simulink model "Code_Gene_Electronic_Throttle_Control_Failure_Model"  (R2024a)
settings: Solver=FixedStepDiscrete  StartTime=0.0  StopTime=10.0  RelTol=1e-3
libraries: simulink x5, SignalEditorBlockLib x2, pil_lib x1
settings Model: Creator=DELL  LastModifiedBy=DELL
settings DataIOCC: ExternalInput=[t, u ]
settings OptimizationCC: DefaultParameterBehavior=Inlined  UseDivisionForNetSlopeComputation=on  GainParamInheritBuiltInType=on  UseFloatMulNetSlope=on  InlineInvariantSignals=on  PassReuseOutputArgsAs=Individual arguments  ZeroExternalMemoryAtStartup=off  ZeroInternalMemoryAtStartup=off  NoFixptDivByZeroProtection=on  EfficientFloat2IntCast=on  LifeSpan=1  OptimizeBlockOrder=speed  DifferentSizesBufferReuse=on  EfficientTunableParamExpr=on
settings DebuggingCC: ParameterTunabilityLossMsg=error
settings HardwareCC: ProdLongLongMode=on
settings SFSimCC: MATLABDynamicMemAlloc=off
settings RTWCC: Description=Embedded Coder  SystemTargetFile=ert.tlc  TemplateMakefile=ert_default_tmf  CreateSILPILBlock=SIL
settings CodeAppCC: ForceParamTrailComments=on  IgnoreCustomStorageClasses=off  OperatorAnnotations=on  SimulinkDataObjDesc=on  SFDataObjDesc=on  CustomSymbolStrGlobalVar=rt$N$M  CustomSymbolStrType=$N$M  CustomSymbolStrFcn=$N$M$F  CustomSymbolStrMacro=$N$M  InsertBlockDesc=on
settings ERTTargetCC: TargetLangStandard=C99 (ISO)  GenerateSampleERTMain=on  IncludeMdlTerminateFcn=off  CombineSignalStateStructs=on  SuppressErrorStatus=on  SupportAbsoluteTime=off  SupportComplex=off  InlinedParameterPlacement=NonHierarchical  ERTCustomFileTemplate=example_file_process.tlc  ERTFilePackagingFormat=CompactWithDataFile

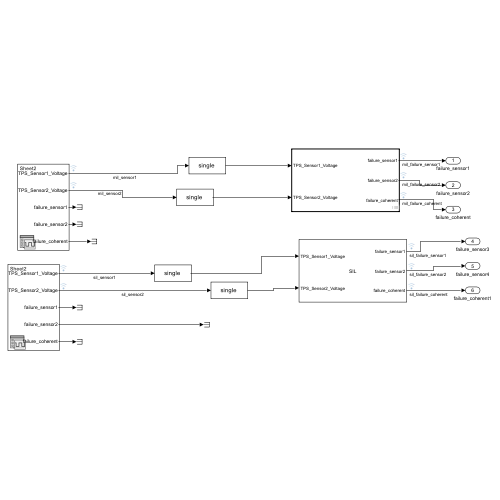
[thumbnail: Simulink's stored preview of the top-level diagram]
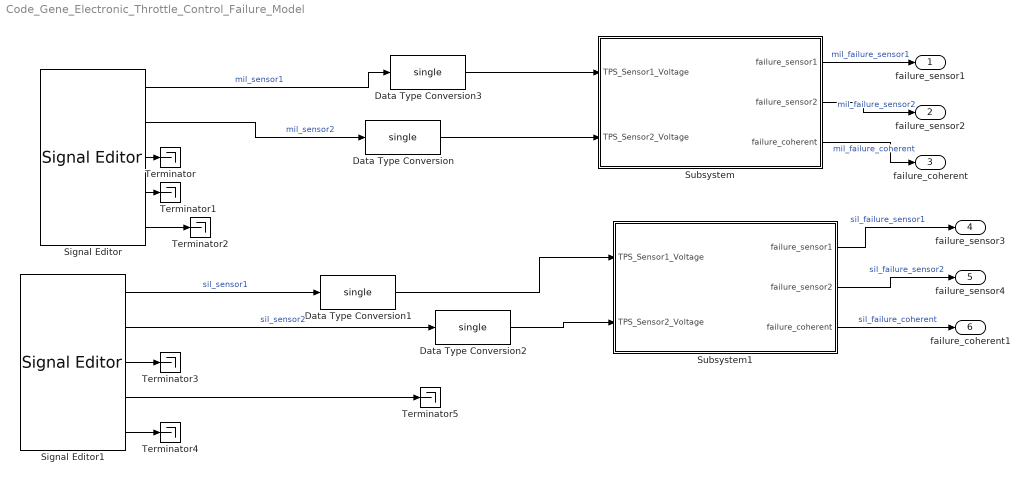
== system Code_Gene_Electronic_Throttle_Control_Failure_Model ==
  Data Type Conversion{,1..3} (4 alike) : DataTypeConversion  OutDataTypeStr=single  SaturateOnIntegerOverflow=off  RndMeth=Floor
  Signal Editor : SignalEditorBlockLib/Signal Editor  FileName=C:\Users\DELL\Desktop\model-based-design\Section9_System_Modelling_Module\tasks\Test_TPS.mat  ActiveScenario=Sheet2  ActiveSignal=TPS_Sensor1_Voltage  IsBus=off  OutputBusObjectStr=Bus: BusObject  SampleTime=0  Interpolate=off  ZeroCross=off  OutputAfterFinalValue=Setting to zero  Unit=inherit  PreserveSignalName=on  ApplySigPropsToAllScenarios=on  ApplySigPropsToAllSignals=off
  Signal Editor1 : SignalEditorBlockLib/Signal Editor  FileName=C:\Users\DELL\Desktop\model-based-design\Section9_System_Modelling_Module\tasks\Test_TPS.mat  ActiveScenario=Sheet2  ActiveSignal=TPS_Sensor1_Voltage  IsBus=off  OutputBusObjectStr=Bus: BusObject  SampleTime=0  Interpolate=off  ZeroCross=off  OutputAfterFinalValue=Setting to zero  Unit=inherit  PreserveSignalName=on  ApplySigPropsToAllScenarios=on  ApplySigPropsToAllSignals=off
  Subsystem : Subsystem  TreatAsAtomicUnit=on
  Subsystem1 : Subsystem  Tag=__SL_testing_harness_stub_  DialogController=pil_create_dialog  LoadFcn=|
      | try
      |    if ~strcmp(rtw.pil.getPILVersion, '24.1 (R2024a)_15')
      |       set_param(gcb, 'DialogController', '');
      |       set_param(gcb, 'DialogControllerArgs', '');
      |    end
      | catch e
      |       set_param(gcb, 'DialogController', '');
      |       set_param(gcb, 'DialogControllerArgs', '');
      | end
      mask help: PIL:pil:XILBlockMaskDesc
      mask Display: disp('SIL');
  Terminator{,1..5} (6 alike) : Terminator
  failure_sensor1 : Outport
  failure_sensor2 : Outport  Port=2
  failure_coherent : Outport  Port=3
  failure_sensor3 : Outport  Port=4
  failure_sensor4 : Outport  Port=5
  failure_coherent1 : Outport  Port=6
  wires:
  Signal Editor/1 -> Data Type Conversion3/1  "mil_sensor1"
  Subsystem/1(failure_sensor1) -> failure_sensor1/1  "mil_failure_sensor1"
  Subsystem/2(failure_sensor2) -> failure_sensor2/1  "mil_failure_sensor2"
  Subsystem/3(failure_coherent) -> failure_coherent/1  "mil_failure_coherent"
  Signal Editor1/1 -> Data Type Conversion1/1  "sil_sensor1"
  Subsystem1/1(failure_sensor1) -> failure_sensor3/1  "sil_failure_sensor1"
  Subsystem1/2(failure_sensor2) -> failure_sensor4/1  "sil_failure_sensor2"
  Subsystem1/3(failure_coherent) -> failure_coherent1/1  "sil_failure_coherent"
  Signal Editor/2 -> Data Type Conversion/1  "mil_sensor2"
  Signal Editor/3 -> Terminator/1
  Signal Editor/4 -> Terminator1/1
  Signal Editor/5 -> Terminator2/1
  Signal Editor1/2 -> Data Type Conversion2/1  "sil_sensor2"
  Signal Editor1/3 -> Terminator3/1
  Signal Editor1/5 -> Terminator4/1
  Signal Editor1/4 -> Terminator5/1
  Data Type Conversion/1 -> Subsystem/2(TPS_Sensor2_Voltage)
  Data Type Conversion1/1 -> Subsystem1/1(TPS_Sensor1_Voltage)
  Data Type Conversion2/1 -> Subsystem1/2(TPS_Sensor2_Voltage)
  Data Type Conversion3/1 -> Subsystem/1(TPS_Sensor1_Voltage)

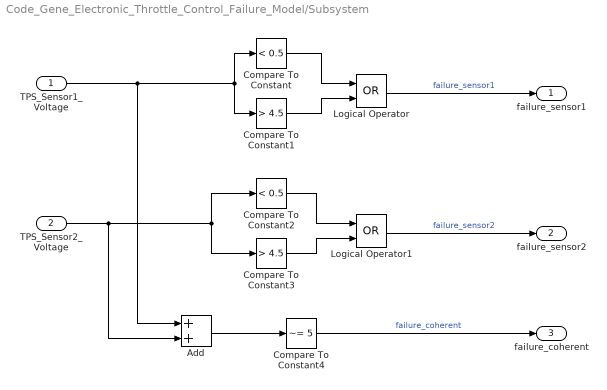
== system Code_Gene_Electronic_Throttle_Control_Failure_Model/Subsystem ==
  TPS_Sensor1_Voltage : Inport  OutDataTypeStr=single
  TPS_Sensor2_Voltage : Inport  Port=2  OutDataTypeStr=single
  Add : Sum
  Compare To Constant : simulink/Logic and Bit Operations/Compare To Constant  relop=<  const=0.5  OutDataTypeStr=boolean
  Compare To Constant1 : simulink/Logic and Bit Operations/Compare To Constant  relop=>  const=4.5  OutDataTypeStr=boolean
  Compare To Constant2 : simulink/Logic and Bit Operations/Compare To Constant  relop=<  const=0.5  OutDataTypeStr=boolean
  Compare To Constant3 : simulink/Logic and Bit Operations/Compare To Constant  relop=>  const=4.5  OutDataTypeStr=boolean  ZeroCross=off
  Compare To Constant4 : simulink/Logic and Bit Operations/Compare To Constant  relop=~=  const=5  OutDataTypeStr=boolean
  Logical Operator : Logic  Operator=OR  AllPortsSameDT=off  OutDataTypeStr=boolean
  Logical Operator1 : Logic  Operator=OR  AllPortsSameDT=off  OutDataTypeStr=boolean
  failure_sensor1 : Outport  OutDataTypeStr=boolean
  failure_sensor2 : Outport  Port=2  OutDataTypeStr=boolean
  failure_coherent : Outport  Port=3  OutDataTypeStr=boolean
  wires:
  Compare To Constant/1 -> Logical Operator/1
  Compare To Constant1/1 -> Logical Operator/2
  Logical Operator/1 -> failure_sensor1/1  "failure_sensor1"
  TPS_Sensor1_Voltage/1 -> Add/1, Compare To Constant/1, Compare To Constant1/1
  TPS_Sensor2_Voltage/1 -> Add/2, Compare To Constant3/1, Compare To Constant2/1
  Compare To Constant2/1 -> Logical Operator1/1
  Compare To Constant3/1 -> Logical Operator1/2
  Logical Operator1/1 -> failure_sensor2/1  "failure_sensor2"
  Add/1 -> Compare To Constant4/1
  Compare To Constant4/1 -> failure_coherent/1  "failure_coherent"

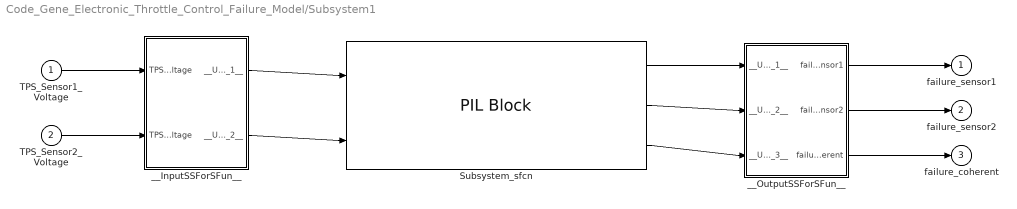
== system Code_Gene_Electronic_Throttle_Control_Failure_Model/Subsystem1 ==
  TPS_Sensor1_Voltage : Inport  OutDataTypeStr=single
  TPS_Sensor2_Voltage : Inport  Port=2  OutDataTypeStr=single
  Subsystem_sfcn : pil_lib/PIL Block  SimulationMode=SIL  IsTopModelPIL=off  CodeDir=Subsystem_ert_rtw  AnchorDir=C:\Users\DELL\Desktop\model-based-design\Section9_System_Modelling_Module\tasks\Code_Gene_Electronic_Throttle_Control_Failure_Model  ConfigName=Software-in-the-Loop (SIL)  XrelIsTopModelCode=on  XrelIsReusable=off  XrelDWorkNames={}  XrelDWorkTypes={}  XrelModelArgVals={}  XrelOrderedParamNames={}  XRelNonFiniteStyle=NONFINITE_UNUSED
  __InputSSForSFun__ : Subsystem
  __OutputSSForSFun__ : Subsystem
  failure_sensor1 : Outport  OutDataTypeStr=boolean
  failure_sensor2 : Outport  Port=2  OutDataTypeStr=boolean
  failure_coherent : Outport  Port=3  OutDataTypeStr=boolean
  wires:
  __OutputSSForSFun__/3(failure_coherent) -> failure_coherent/1
  __OutputSSForSFun__/2(failure_sensor2) -> failure_sensor2/1
  __OutputSSForSFun__/1(failure_sensor1) -> failure_sensor1/1
  Subsystem_sfcn/3 -> __OutputSSForSFun__/3(__UniqueInportName__3__)
  Subsystem_sfcn/2 -> __OutputSSForSFun__/2(__UniqueInportName__2__)
  Subsystem_sfcn/1 -> __OutputSSForSFun__/1(__UniqueInportName__1__)
  __InputSSForSFun__/2(__UniqueOutportName__2__) -> Subsystem_sfcn/2
  __InputSSForSFun__/1(__UniqueOutportName__1__) -> Subsystem_sfcn/1
  TPS_Sensor2_Voltage/1 -> __InputSSForSFun__/2(TPS_Sensor2_Voltage)
  TPS_Sensor1_Voltage/1 -> __InputSSForSFun__/1(TPS_Sensor1_Voltage)

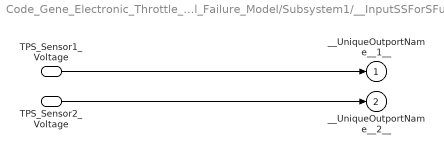
== system Code_Gene_Electronic_Throttle_Control_Failure_Model/Subsystem1/__InputSSForSFun__ ==
  TPS_Sensor1_Voltage : Inport  OutDataTypeStr=single
  TPS_Sensor2_Voltage : Inport  Port=2  OutDataTypeStr=single
  __UniqueOutportName__1__ : Outport
  __UniqueOutportName__2__ : Outport  Port=2
  wires:
  TPS_Sensor2_Voltage/1 -> __UniqueOutportName__2__/1
  TPS_Sensor1_Voltage/1 -> __UniqueOutportName__1__/1

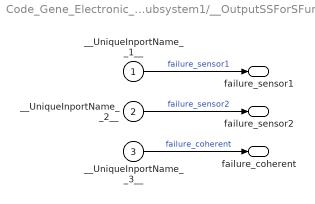
== system Code_Gene_Electronic_Throttle_Control_Failure_Model/Subsystem1/__OutputSSForSFun__ ==
  __UniqueInportName__1__ : Inport
  __UniqueInportName__2__ : Inport  Port=2
  __UniqueInportName__3__ : Inport  Port=3
  failure_sensor1 : Outport  OutDataTypeStr=boolean
  failure_sensor2 : Outport  Port=2  OutDataTypeStr=boolean
  failure_coherent : Outport  Port=3  OutDataTypeStr=boolean
  wires:
  __UniqueInportName__3__/1 -> failure_coherent/1  "failure_coherent"
  __UniqueInportName__2__/1 -> failure_sensor2/1  "failure_sensor2"
  __UniqueInportName__1__/1 -> failure_sensor1/1  "failure_sensor1"
